simulink model "satBFrob2_v2017"  (R2017b)
settings: Solver=VariableStepAuto  StartTime=0.0  StopTime=100.0  RelTol=1e-3
settings Model: Creator=t.lopes  LastModifiedBy=xylow

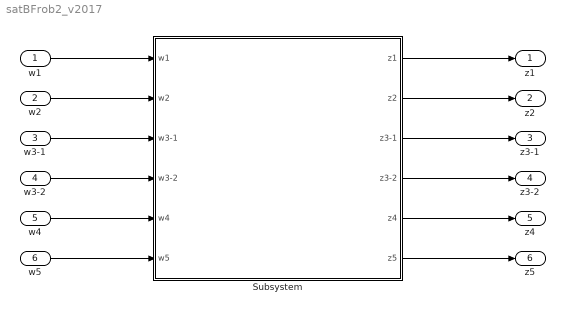
== system satBFrob2_v2017 ==
  w1 : Inport
  "w2 " : Inport  Port=2
  w3-1 : Inport  Port=3
  w3-2 : Inport  Port=4
  w4 : Inport  Port=5
  w5 : Inport  Port=6
  Subsystem : Subsystem
  z1 : Outport
  z2 : Outport  Port=2
  z3-1 : Outport  Port=3
  z3-2 : Outport  Port=4
  z4 : Outport  Port=5
  z5 : Outport  Port=6
  wires:
  w3-1/1 -> Subsystem/3(w3-1)
  w4/1 -> Subsystem/5(w4)
  w5/1 -> Subsystem/6(w5)
  w3-2/1 -> Subsystem/4(w3-2)
  Subsystem/3(z3-1) -> z3-1/1
  Subsystem/6(z5) -> z5/1
  Subsystem/4(z3-2) -> z3-2/1
  Subsystem/5(z4) -> z4/1
  w1/1 -> Subsystem/1(w1)
  "w2 "/1 -> Subsystem/2(w2)
  Subsystem/1(z1) -> z1/1
  Subsystem/2(z2) -> z2/1

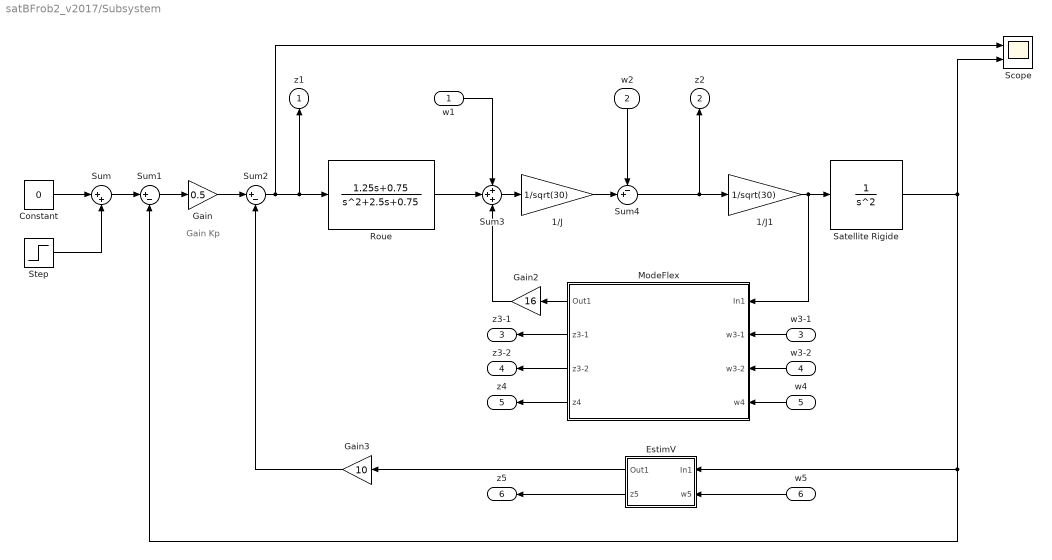
== system satBFrob2_v2017/Subsystem ==
  note: Gain Kp
  w1 : Inport
  w2 : Inport  Port=2
  w3-1 : Inport  Port=3
  w3-2 : Inport  Port=4
  w4 : Inport  Port=5
  w5 : Inport  Port=6
  1/J : Gain  Gain=1/sqrt(30)
  1/J1 : Gain  Gain=1/sqrt(30)
  Constant : Constant  Value=0
  EstimV : Subsystem
  Gain : Gain  Gain=0.5
  Gain2 : Gain  Gain=16
  Gain3 : Gain  Gain=10
  ModeFlex : Subsystem
  Roue : TransferFcn  Numerator=[1.25 0.75]  Denominator=[1 2.5 0.75]
  Satellite Rigide : TransferFcn  Denominator=[1 0 0]
  Scope : Scope  NumInputPorts=2
  Step : Step  SampleTime=0
  Sum : Sum  Inputs=|++
  Sum1 : Sum  Inputs=|+-
  Sum2 : Sum  Inputs=|+-
  Sum3 : Sum  Inputs=+++
  Sum4 : Sum  Inputs=-+|
  z1 : Outport
  z2 : Outport  Port=2
  z3-1 : Outport  Port=3
  z3-2 : Outport  Port=4
  z4 : Outport  Port=5
  z5 : Outport  Port=6
  wires:
  ModeFlex/4(z4) -> z4/1
  1/J/1 -> Sum4/2
  Sum/1 -> Sum1/1
  ModeFlex/2(z3-1) -> z3-1/1
  w3-2/1 -> ModeFlex/3(w3-2)
  w4/1 -> ModeFlex/4(w4)
  Gain2/1 -> Sum3/3
  Gain3/1 -> Sum2/2
  Roue/1 -> Sum3/2
  Satellite Rigide/1 -> Scope/2, Sum1/2, EstimV/1(In1)
  EstimV/1(Out1) -> Gain3/1
  Step/1 -> Sum/2
  Sum2/1 -> Scope/1, z1/1, Roue/1
  1/J1/1 -> ModeFlex/1(In1), Satellite Rigide/1
  w2/1 -> Sum4/1
  Sum4/1 -> z2/1, 1/J1/1
  ModeFlex/1(Out1) -> Gain2/1
  Gain/1 -> Sum2/1
  w5/1 -> EstimV/2(w5)
  ModeFlex/3(z3-2) -> z3-2/1
  EstimV/2(z5) -> z5/1
  w3-1/1 -> ModeFlex/2(w3-1)
  w1/1 -> Sum3/1
  Sum3/1 -> 1/J/1
  Sum1/1 -> Gain/1
  Constant/1 -> Sum/1

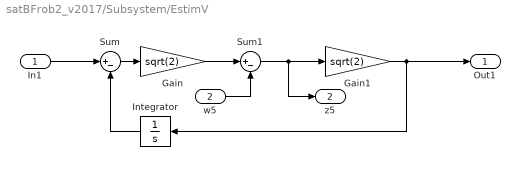
== system satBFrob2_v2017/Subsystem/EstimV ==
  In1 : Inport
  w5 : Inport  Port=2
  Gain : Gain  Gain=sqrt(2)
  Gain1 : Gain  Gain=sqrt(2)
  Integrator : Integrator
  Sum : Sum  Inputs=|+-
  Sum1 : Sum  Inputs=|+-
  Out1 : Outport
  z5 : Outport  Port=2
  wires:
  Sum/1 -> Gain/1
  Integrator/1 -> Sum/2
  In1/1 -> Sum/1
  Gain/1 -> Sum1/1
  w5/1 -> Sum1/2
  Sum1/1 -> z5/1, Gain1/1
  Gain1/1 -> Integrator/1, Out1/1

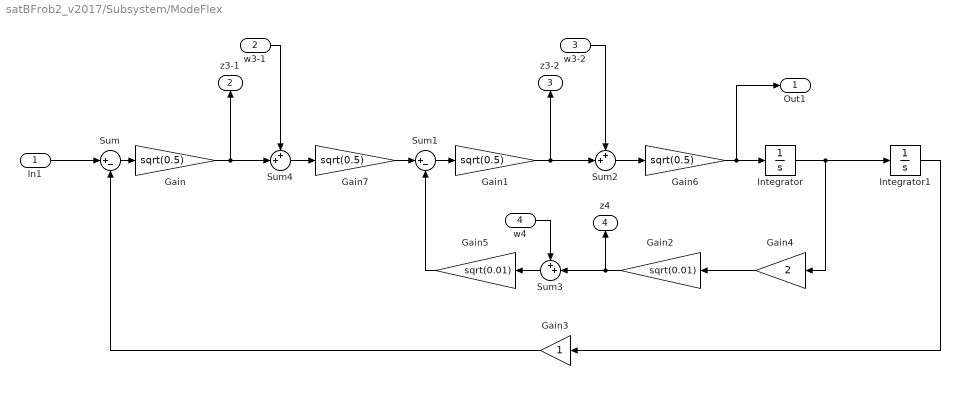
== system satBFrob2_v2017/Subsystem/ModeFlex ==
  In1 : Inport
  w3-1 : Inport  Port=2
  w3-2 : Inport  Port=3
  w4 : Inport  Port=4
  Gain{,1,6..7} (4 alike) : Gain  Gain=sqrt(0.5)
  Gain2 : Gain  Gain=sqrt(0.01)
  Gain3 : Gain
  Gain4 : Gain  Gain=2
  Gain5 : Gain  Gain=sqrt(0.01)
  Integrator : Integrator
  Integrator1 : Integrator
  Sum : Sum  Inputs=|+-
  Sum1 : Sum  Inputs=|+-
  Sum2 : Sum  Inputs=++|
  Sum3 : Sum  Inputs=++|
  Sum4 : Sum  Inputs=++|
  Out1 : Outport
  z3-1 : Outport  Port=2
  z3-2 : Outport  Port=3
  z4 : Outport  Port=4
  wires:
  In1/1 -> Sum/1
  Sum/1 -> Gain/1
  Sum1/1 -> Gain1/1
  Gain1/1 -> z3-2/1, Sum2/2
  Integrator1/1 -> Gain3/1
  Integrator/1 -> Gain4/1, Integrator1/1
  Gain3/1 -> Sum/2
  Gain4/1 -> Gain2/1
  w3-1/1 -> Sum4/1
  Gain/1 -> Sum4/2, z3-1/1
  w3-2/1 -> Sum2/1
  Gain2/1 -> z4/1, Sum3/2
  Sum3/1 -> Gain5/1
  w4/1 -> Sum3/1
  Gain5/1 -> Sum1/2
  Sum2/1 -> Gain6/1
  Gain6/1 -> Out1/1, Integrator/1
  Sum4/1 -> Gain7/1
  Gain7/1 -> Sum1/1
